simulink model "targetingLib"  (R2026b)
settings: Solver=VariableStepAuto
undefined symbols (not defined in the file or in its folder): maxval_sc, minval_sc, modval, samptime, Slope1, Slope2, threshold_add
libraries: hdlsllib x57, simulink x19, simulink_extras x11, dspsigops x2, sl_signal_attributes x2
(part 2 of 3)

== system targetingLib/Energy Detector/CalibrationPacketisation/Detect Overflow1 ==
  note: Throw away if not ready.
      | Assume will always be ready due to low rates.
  Ready : Inport
  Valid : Inport  Port=2
  EOB : Inport  Port=3
  AND1 : Logic  IconShape=distinctive  AllPortsSameDT=off  OutDataTypeStr=boolean
  AND2 : Logic  IconShape=distinctive  AllPortsSameDT=off  OutDataTypeStr=boolean
  Delay : Delay  DelayLength=1
  NOT : Logic  Operator=NOT  IconShape=distinctive  AllPortsSameDT=off  OutDataTypeStr=boolean
  Reset on next burst : simulink_extras/Flip Flops/S-R Flip-Flop  initial_condition=0
  Start of Burst : Subsystem
  Terminator : Terminator
  ValidOut : Outport
  OverflowOut : Outport  Port=2
  wires:
  AND1/1 -> ValidOut/1
  Ready/1 -> AND1/2, NOT/1
  Valid/1 -> AND2/2, Start of Burst/1(Valid), AND1/1  "Valid"
  NOT/1 -> AND2/1
  EOB/1 -> Start of Burst/2(EOB)  "EOB"
  Start of Burst/1(SOB) -> Reset on next burst/2
  AND2/1 -> Delay/1
  Reset on next burst/1 -> OverflowOut/1
  Reset on next burst/2 -> Terminator/1
  Delay/1 -> Reset on next burst/1

== system targetingLib/Energy Detector/Detect Overflow/Start of Burst ==
  Valid : Inport
  EOB : Inport  Port=2
  Detect Increase : simulink/Logic and Bit Operations/Detect Increase  vinit=0.0  OutDataTypeStr=boolean
  S-R Flip-Flop : simulink_extras/Flip Flops/S-R Flip-Flop  initial_condition=0
  Terminator : Terminator
  SOB : Outport
  wires:
  S-R Flip-Flop/1 -> Detect Increase/1
  EOB/1 -> S-R Flip-Flop/2
  S-R Flip-Flop/2 -> Terminator/1
  Detect Increase/1 -> SOB/1  "SOB"
  Valid/1 -> S-R Flip-Flop/1

== system targetingLib/Energy Detector/Energy Detector/Create Meta Data Stream ==
  note: 16 bits of pulse count
  note: Save pulse detection metadata as a uint32
  note: 16 bits of peak energy
  Energy : Inport
  Triggered_Data_Bus_Out : Inport  Port=2
  AND : Logic  IconShape=distinctive  AllPortsSameDT=off  OutDataTypeStr=boolean
  Bit Concat : hdlsllib/Logic and Bit Operations/Bit Concat  numInputs=2
  Bit Slice : hdlsllib/Logic and Bit Operations/Bit Slice  lidx=31  ridx=0
  Bit Slice1 : hdlsllib/Logic and Bit Operations/Bit Slice  lidx=63  ridx=32
  Bus Selector1 : BusSelector  OutputSignals=valid
  Bus Selector2 : BusSelector  OutputSignals=sampleTimestamp
  Bus Selector3 : BusSelector  OutputSignals=EndOfBurst
  Compare To Constant : simulink/Logic and Bit Operations/Compare To Constant  relop===  const=0  OutDataTypeStr=boolean
  Delay1 : Delay  DelayLength=1
  Delay2 : Delay  DelayLength=1
  Delay3 : Delay
  Delay4 : Delay  DelayLength=1
  Detect Increase : simulink/Logic and Bit Operations/Detect Increase  vinit=0.0  OutDataTypeStr=boolean
  Detected Pulse Length Counter : Subsystem
  Float Typecast1 : FloatTypecast
  Multiport Switch : MultiPortSwitch  DataPortOrder=Zero-based contiguous  zeroidx=on  SaturateOnIntegerOverflow=off  InputSameDT=off
  Multiport Controller : Subsystem
  Peak pulse energy : Subsystem
  Meta_Data_Data : Outport
  Meta_Data_Valid : Outport  Port=2
  wires:
  Triggered_Data_Bus_Out/1 -> Bus Selector3/1, Bus Selector1/1, Bus Selector2/1
  Energy/1 -> Peak pulse energy/1(energy)
  Float Typecast1/1 -> Bit Concat/1
  Bus Selector3/1 -> Detect Increase/1  "<EndOfBurst>"
  Detected Pulse Length Counter/1(count) -> Bit Concat/2
  Peak pulse energy/1(peak) -> Float Typecast1/1
  Detect Increase/1 -> Delay2/1
  Bus Selector1/1 -> Peak pulse energy/3(valid), Detected Pulse Length Counter/2(valid)  "<valid>"
  Bus Selector2/1 -> Bit Slice1/1, Bit Slice/1  "<sampleTimestamp>"
  Multiport Switch/1 -> Meta_Data_Data/1
  Bit Concat/1 -> Multiport Switch/2
  Bit Slice1/1 -> Delay1/1
  Bit Slice/1 -> Delay3/1
  Delay1/1 -> Multiport Switch/3
  Delay3/1 -> Multiport Switch/4
  Delay2/1 -> Multiport Controller/1(EoB_Asserted)
  Multiport Controller/2(count) -> Compare To Constant/1, Multiport Switch/1
  Multiport Controller/1(valid_out) -> AND/2, Meta_Data_Valid/1
  [PeakRst] -> Detected Pulse Length Counter/1(rst), Peak pulse energy/2(rst)
  Compare To Constant/1 -> AND/1
  AND/1 -> Delay4/1
  Delay4/1 -> [PeakRst]

== system targetingLib/Energy Detector/Energy Detector/Energy Detector ==
  DataBusIn : Inport
  WindowLength : Inport  Port=2
  AdaptiveThreshold : Inport  Port=3
  AdaptiveEndThreshold : Inport  Port=4
  AdaptiveThresholdScaler : Inport  Port=5
  FixedThreshold : Inport  Port=6
  Bus Selector : BusSelector  OutputSignals=EndOfBurst
  Delay : Delay  DelayLength=1
  Signal Detection : Subsystem
  Energy : Outport
  DataBusOut : Outport  Port=2
  Triggered : Outport  Port=3
  CalibrationOut : Outport  Port=4
  wires:
  WindowLength/1 -> Signal Detection/3(delay_len)  "WindowLength"
  FixedThreshold/1 -> Signal Detection/4(fix_threshold_in)  "FixedThreshold"
  DataBusIn/1 -> Signal Detection/2(data_bus_in)
  Signal Detection/3(Trigger_Out) -> Triggered/1
  Signal Detection/4(Energy_out) -> Energy/1
  Signal Detection/2(FT_Data_Out) -> CalibrationOut/1
  Delay/1 -> Signal Detection/1(rst)
  Signal Detection/1(Data_Bus_Out) -> Bus Selector/1, DataBusOut/1
  AdaptiveThreshold/1 -> Signal Detection/5(adp_threshold_in)  "AdaptiveThreshold"
  AdaptiveThresholdScaler/1 -> Signal Detection/7(adp_normalizer)  "AdaptiveThresholdScaler"
  AdaptiveEndThreshold/1 -> Signal Detection/6(adp_end_threshold_in)  "AdaptiveEndThreshold"
  Bus Selector/1 -> Delay/1  "<EndOfBurst>"

== system targetingLib/Energy Detector/Energy Detector/Triggered Burst Formatting ==
  note: Reset state when Burst from Radio ends (EOB from Radio)
  note: Handle trigger not in sync with Valid by holding EOB high
  note: When data is valid and trigger is true, out is valid
  note: Trigger is de-asserted, end the burst.
  Data_Bus_In : Inport
  Trigger : Inport  Port=2
  AND : Logic  IconShape=distinctive  AllPortsSameDT=off  OutDataTypeStr=boolean
  AND1 : Logic  IconShape=distinctive  AllPortsSameDT=off  OutDataTypeStr=boolean
  Bus Selector : BusSelector  OutputSignals=data,sampleTimestamp,valid,EndOfBurst
  Bus Selector1 : BusSelector  OutputSignals=data,sampleTimestamp
  Data Bus : BusCreator  Inputs=4
  Delay1 : Delay
  Delay2 : Delay
  Delay3 : Delay  DelayLength=1
  Delay4 : Delay  DelayLength=1
  Delay5 : Delay
  End of trigger : simulink/Logic and Bit Operations/Detect Decrease  vinit=0.0  OutDataTypeStr=boolean
  EndedByRadio : Logic  IconShape=distinctive  AllPortsSameDT=off  OutDataTypeStr=boolean
  OR : Logic  Operator=OR  IconShape=distinctive  AllPortsSameDT=off  OutDataTypeStr=boolean
  S-R Flip-Flop : simulink_extras/Flip Flops/S-R Flip-Flop  initial_condition=0
  Sideband Bus : BusCreator  Inputs=2
  Terminator : Terminator
  Data_Bus_Out : Outport
  Reset_Out : Outport  Port=2
  wires:
  Trigger/1 -> EndedByRadio/1, End of trigger/1, AND/1
  AND/1 -> Delay1/1
  End of trigger/1 -> OR/1
  Delay1/1 -> Data Bus/3, AND1/1  "valid"
  OR/1 -> Delay4/1
  S-R Flip-Flop/1 -> AND1/2, Data Bus/4  "EndOfBurst"
  AND1/1 -> Delay3/1
  S-R Flip-Flop/2 -> Terminator/1
  Delay3/1 -> S-R Flip-Flop/2
  Delay4/1 -> S-R Flip-Flop/1
  Delay5/1 -> Reset_Out/1
  Data_Bus_In/1 -> Bus Selector/1
  Bus Selector/3 -> AND/2  "<valid>"
  Bus Selector/4 -> Delay5/1, EndedByRadio/2  "<EndOfBurst>"
  Bus Selector/1 -> Sideband Bus/1  "<data>"
  Bus Selector/2 -> Sideband Bus/2  "<sampleTimestamp>"
  Sideband Bus/1 -> Delay2/1  "SidebandBus"
  Delay2/1 -> Bus Selector1/1
  Bus Selector1/1 -> Data Bus/1  "<data>"
  Bus Selector1/2 -> Data Bus/2  "<sampleTimestamp>"
  Data Bus/1 -> Data_Bus_Out/1
  EndedByRadio/1 -> OR/2

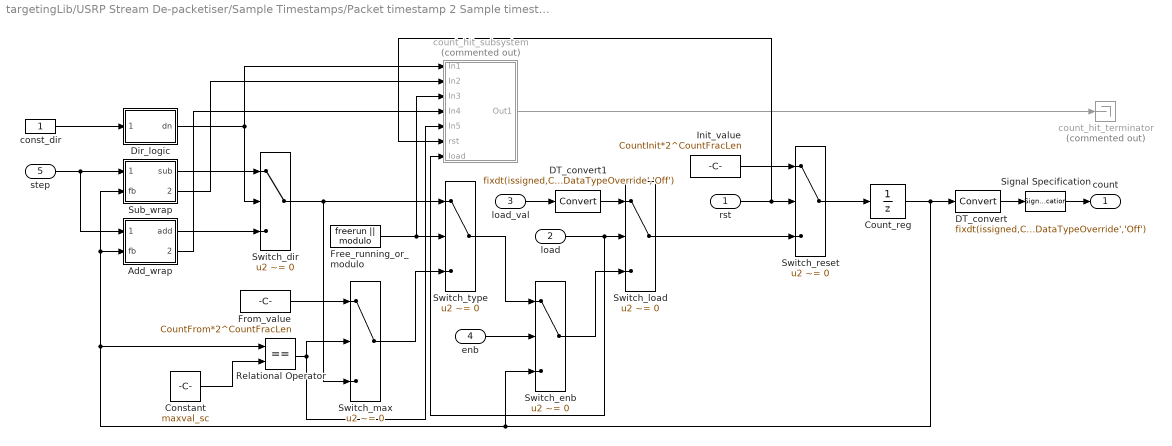
== system targetingLib/USRP Stream De-packetiser/Sample Timestamps/Packet timestamp 2 Sample timestamp ==
  rst : Inport  OutDataTypeStr=boolean  PortDimensions=1
  load : Inport  Port=2  OutDataTypeStr=boolean  PortDimensions=1
  load_val : Inport  Port=3  OutDataTypeStr=fixdt(issigned,CountWordLen,CountFracLen,'DataTypeOverride','Off')  PortDimensions=1
  enb : Inport  Port=4  OutDataTypeStr=boolean  PortDimensions=1
  step : Inport  Port=5  OutDataTypeStr=uint64  PortDimensions=1
  Add_wrap : Subsystem
  Constant : Constant  Value=maxval_sc  OutDataTypeStr=fixdt(issigned,CountWordLen,0,'DataTypeOverride','Off')  SampleTime=-1
  Count_reg : UnitDelay  InitialCondition=CountInit*2^CountFracLen  SampleTime=samptime
  DT_convert : DataTypeConversion  OutDataTypeStr=fixdt(issigned,CountWordLen,CountFracLen,'DataTypeOverride','Off')  ConvertRealWorld=Stored Integer (SI)  SaturateOnIntegerOverflow=off  RndMeth=Floor
  DT_convert1 : DataTypeConversion  OutDataTypeStr=fixdt(issigned,CountWordLen,0,'DataTypeOverride','Off')  ConvertRealWorld=Stored Integer (SI)  SaturateOnIntegerOverflow=off  RndMeth=Floor
  Dir_logic : Subsystem
  Free_running_or_modulo : Constant  Value=freerun || modulo  OutDataTypeStr=boolean  SampleTime=-1
  From_value : Constant  Value=CountFrom*2^CountFracLen  OutDataTypeStr=fixdt(issigned,CountWordLen, 0,'DataTypeOverride','Off')  SampleTime=-1
  Init_value : Constant  Value=CountInit*2^CountFracLen  OutDataTypeStr=fixdt(issigned,CountWordLen, 0,'DataTypeOverride','Off')  SampleTime=-1
  Relational Operator : RelationalOperator  Operator===  OutDataTypeStr=boolean  RndMeth=Simplest  InputSameDT=off
  Signal Specification : SignalSpecification  Dimensions=1
  Sub_wrap : Subsystem
  Switch_dir : Switch  Criteria=u2 ~= 0  SaturateOnIntegerOverflow=off  InputSameDT=off
  Switch_enb : Switch  Criteria=u2 ~= 0  SaturateOnIntegerOverflow=off  InputSameDT=off
  Switch_load : Switch  Criteria=u2 ~= 0  SaturateOnIntegerOverflow=off  InputSameDT=off
  Switch_max : Switch  Criteria=u2 ~= 0  SaturateOnIntegerOverflow=off  InputSameDT=off
  Switch_reset : Switch  Criteria=u2 ~= 0  OutDataTypeStr=fixdt(issigned,CountWordLen, 0,'DataTypeOverride','Off')  SaturateOnIntegerOverflow=off  InputSameDT=off
  Switch_type : Switch  Criteria=u2 ~= 0  SaturateOnIntegerOverflow=off  InputSameDT=off
  const_dir : Constant  OutDataTypeStr=boolean  SampleTime=-1
  count_hit_subsystem : Subsystem  Commented=on
  count_hit_terminator : Terminator  Commented=on
  count : Outport  OutDataTypeStr=uint64  VectorParamsAs1DForOutWhenUnconnected=off
  wires:
  count_hit_subsystem/1(Out1) -> count_hit_terminator/1
  Add_wrap/2(count_hit) -> count_hit_subsystem/4(In4)
  Sub_wrap/2(count_hit) -> count_hit_subsystem/2(In2)
  Relational Operator/1 -> count_hit_subsystem/5(In5), Switch_max/2
  Constant/1 -> Relational Operator/2
  Switch_dir/1 -> Switch_type/1, Switch_max/3
  Init_value/1 -> Switch_reset/1
  rst/1 -> Switch_reset/2, count_hit_subsystem/6(rst)
  Switch_reset/1 -> Count_reg/1
  Count_reg/1 -> Switch_enb/3, Sub_wrap/2(fb), Add_wrap/2(fb), Relational Operator/1, DT_convert/1
  Switch_load/1 -> Switch_reset/3
  load/1 -> Switch_load/2, count_hit_subsystem/7(load)
  load_val/1 -> DT_convert1/1
  Switch_enb/1 -> Switch_load/3
  enb/1 -> Switch_enb/2
  const_dir/1 -> Dir_logic/1(dir_port)
  step/1 -> Add_wrap/1(step), Sub_wrap/1(step)
  Switch_type/1 -> Switch_enb/1
  From_value/1 -> Switch_max/1
  Switch_max/1 -> Switch_type/3
  Free_running_or_modulo/1 -> Switch_type/2, count_hit_subsystem/3(In3)
  DT_convert/1 -> Signal Specification/1
  Add_wrap/1(add) -> Switch_dir/3
  Sub_wrap/1(sub) -> Switch_dir/1
  Dir_logic/1(dn) -> Switch_dir/2, count_hit_subsystem/1(In1)
  DT_convert1/1 -> Switch_load/1
  Signal Specification/1 -> count/1

== system targetingLib/Energy Detector/CalibrationPacketisation/Detect Overflow/Start of Burst ==
  Valid : Inport
  EOB : Inport  Port=2
  Detect Increase : simulink/Logic and Bit Operations/Detect Increase  vinit=0.0  OutDataTypeStr=boolean
  S-R Flip-Flop : simulink_extras/Flip Flops/S-R Flip-Flop  initial_condition=0
  Terminator : Terminator
  SOB : Outport
  wires:
  S-R Flip-Flop/1 -> Detect Increase/1
  EOB/1 -> S-R Flip-Flop/2
  S-R Flip-Flop/2 -> Terminator/1
  Detect Increase/1 -> SOB/1  "SOB"
  Valid/1 -> S-R Flip-Flop/1

== system targetingLib/Energy Detector/CalibrationPacketisation/Detect Overflow1/Start of Burst ==
  Valid : Inport
  EOB : Inport  Port=2
  Detect Increase : simulink/Logic and Bit Operations/Detect Increase  vinit=0.0  OutDataTypeStr=boolean
  S-R Flip-Flop : simulink_extras/Flip Flops/S-R Flip-Flop  initial_condition=0
  Terminator : Terminator
  SOB : Outport
  wires:
  S-R Flip-Flop/1 -> Detect Increase/1
  EOB/1 -> S-R Flip-Flop/2
  S-R Flip-Flop/2 -> Terminator/1
  Detect Increase/1 -> SOB/1  "SOB"
  Valid/1 -> S-R Flip-Flop/1

== system targetingLib/Energy Detector/Energy Detector/Create Meta Data Stream/Detected Pulse Length Counter ==
  note: when overflow, set count to zero
  rst : Inport
  valid : Inport  Port=2
  Constant : Constant  Value=0  OutDataTypeStr=Inherit: Inherit via back propagation
  HDL Counter : hdlsllib/Sources/HDL Counter  CountType=Free running  CountInit=0  CountStep=1  CountMax=25  CountFromType=Initial value  CountFrom=0  CountResetPort=on  CountLoadPort=off  CountEnbPort=on  CountDirPort=off  CountHitOutputPort=on  CountDataType=Unsigned  CountWordLen=16  CountFracLen=0  CountSampTime=1
  Multiport Switch : MultiPortSwitch  DataPortOrder=Zero-based contiguous  Inputs=2  zeroidx=on  SaturateOnIntegerOverflow=off  InputSameDT=off
  S-R Flip-Flop : simulink_extras/Flip Flops/S-R Flip-Flop  initial_condition=0
  Terminator : Terminator
  count : Outport
  wires:
  valid/1 -> HDL Counter/2
  HDL Counter/2 -> S-R Flip-Flop/1
  rst/1 -> S-R Flip-Flop/2, HDL Counter/1
  S-R Flip-Flop/2 -> Terminator/1
  S-R Flip-Flop/1 -> Multiport Switch/1
  HDL Counter/1 -> Multiport Switch/2
  Constant/1 -> Multiport Switch/3
  Multiport Switch/1 -> count/1

== system targetingLib/Energy Detector/Energy Detector/Create Meta Data Stream/Multiport Controller ==
  note: On EoB (end of detected pulse), hold metadata valid high for three cycles and iterate the multiport switch index
  EoB_Asserted : Inport
  Delay : Delay  DelayLength=1  InputProcessing=Columns as channels (frame based)
  HDL Counter : hdlsllib/Sources/HDL Counter  CountType=Count limited  CountInit=0  CountStep=1  CountMax=2  CountFromType=Initial value  CountFrom=0  CountResetPort=off  CountLoadPort=off  CountEnbPort=on  CountDirPort=off  CountHitOutputPort=on  CountDataType=Unsigned  CountWordLen=2  CountFracLen=0  CountSampTime=1
  S-R Flip-Flop : simulink_extras/Flip Flops/S-R Flip-Flop  initial_condition=0
  Terminator : Terminator
  valid_out : Outport
  count : Outport  Port=2
  wires:
  HDL Counter/2 -> Delay/1
  S-R Flip-Flop/1 -> valid_out/1, HDL Counter/1
  S-R Flip-Flop/2 -> Terminator/1
  EoB_Asserted/1 -> S-R Flip-Flop/1
  HDL Counter/1 -> count/1
  Delay/1 -> S-R Flip-Flop/2

== system targetingLib/Energy Detector/Energy Detector/Create Meta Data Stream/Peak pulse energy ==
  energy : Inport
  rst : Inport  Port=2
  valid : Inport  Port=3
  AND : Logic  Inputs=3  IconShape=distinctive  AllPortsSameDT=off  OutDataTypeStr=boolean
  AND1 : Logic  IconShape=distinctive  AllPortsSameDT=off  OutDataTypeStr=boolean
  Constant : Constant  Value=0  OutDataTypeStr=Inherit: Inherit via back propagation
  Delay{1..3,5} (4 alike) : Delay  DelayLength=1
  GreaterThan : RelationalOperator  Operator=>  OutDataTypeStr=boolean  RndMeth=Simplest  InputSameDT=off
  GreaterThan1 : RelationalOperator  Operator=>  OutDataTypeStr=boolean  RndMeth=Simplest  InputSameDT=off
  Multiport Switch : MultiPortSwitch  DataPortOrder=Zero-based contiguous  Inputs=2  zeroidx=on  SaturateOnIntegerOverflow=off  InputSameDT=off
  NOT : Logic  Operator=NOT  IconShape=distinctive  AllPortsSameDT=off  OutDataTypeStr=boolean
  NOT1 : Logic  Operator=NOT  IconShape=distinctive  AllPortsSameDT=off  OutDataTypeStr=boolean
  OR : Logic  Operator=OR  IconShape=distinctive  AllPortsSameDT=off  OutDataTypeStr=boolean
  Sample and Hold : dspsigops/Sample and Hold  trig=Falling edge  initCond=0  latchinput=off
  peak : Outport
  wires:
  Sample and Hold/1 -> Delay1/1, peak/1  "Held_Peak_Energy"
  rst/1 -> NOT/1, Delay2/1
  energy/1 -> Multiport Switch/3
  Constant/1 -> Multiport Switch/2
  OR/1 -> Delay5/1
  Delay1/1 -> GreaterThan/2
  valid/1 -> AND/3
  AND/1 -> Multiport Switch/1
  NOT/1 -> AND/2
  NOT1/1 -> AND/1
  Multiport Switch/1 -> Delay3/1, GreaterThan/1, GreaterThan1/1  "S&H_In_z-1"
  Delay2/1 -> OR/1, NOT1/1
  Delay5/1 -> Sample and Hold/Trigger  "S&H_Trigger"
  Delay3/1 -> GreaterThan1/2, Sample and Hold/1  "S&H_In"
  GreaterThan/1 -> AND1/1
  AND1/1 -> OR/2
  GreaterThan1/1 -> AND1/2

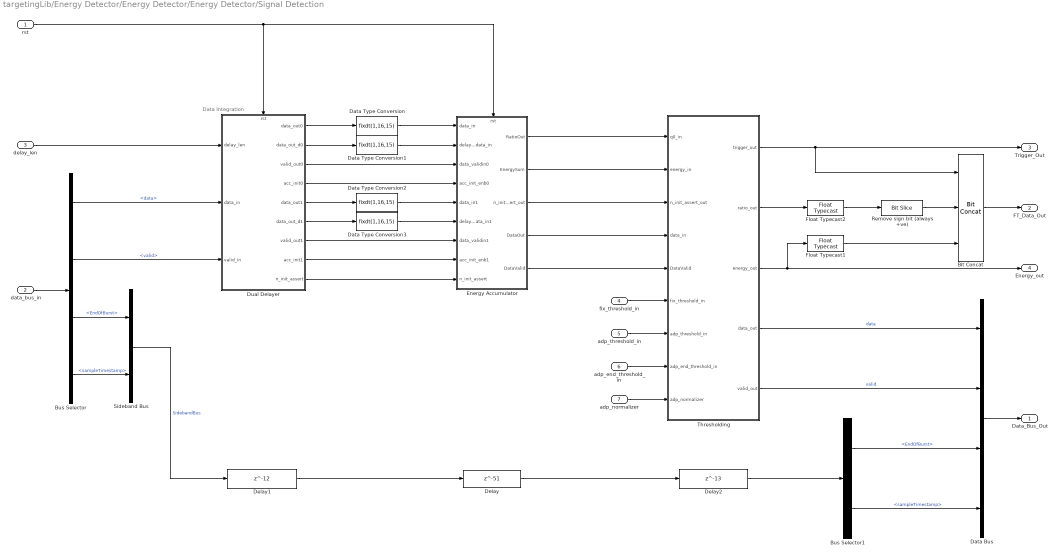
== system targetingLib/Energy Detector/Energy Detector/Energy Detector/Signal Detection ==
  note: Data Integration
  rst : Inport
  data_bus_in : Inport  Port=2
  delay_len : Inport  Port=3
  fix_threshold_in : Inport  Port=4
  adp_threshold_in : Inport  Port=5
  adp_end_threshold_in : Inport  Port=6
  adp_normalizer : Inport  Port=7
  Bit Concat : hdlsllib/Logic and Bit Operations/Bit Concat  numInputs=3
  Bus Selector : BusSelector  OutputSignals=data,valid,EndOfBurst,sampleTimestamp
  Bus Selector1 : BusSelector  OutputSignals=EndOfBurst,sampleTimestamp
  Data Bus : BusCreator  Inputs=4
  Data Type Conversion{,1..3} (4 alike) : DataTypeConversion  OutDataTypeStr=fixdt(1,16,15)  ConvertRealWorld=Stored Integer (SI)  SaturateOnIntegerOverflow=off  RndMeth=Floor
  Delay : Delay  DelayLength=51
  Delay1 : Delay  DelayLength=12
  Delay2 : Delay  DelayLength=13
  Dual Delayer : Subsystem
      settings: PortSchema="{\"entries\":[{\"content\":{\"sides\":[{\"content\":{\"connectorIds\":[\"In1\",\"In2\",\"In3\"]},\"type\":\"ConnectorPlacement.EquallySpacedRectSide\",\"uuid\":\"1990f724-ce81-4930-8303-ca4574d8597a\"},{\"content\":{\"connectorIds\":[\"Out1\",\"Out2\",\"Out3\",\"Out4\",\"Out5\",\"Out6\",\"Out7\",\"Out8\",\"Out9\"],\"side\":\"RIGHT\"},\"type\":\"ConnectorPlacement.EquallySpacedRectSide\",\"uuid\":\"07aa7081-9df9-4b7b-99cf-18a69e24a9dd\"},{\"content\":{\"connectorIds\":[\"In4\"],\"side\":\"TOP\"},\"type\":\"ConnectorPlacement.EquallySpacedRectSide\",\"uuid\":\"c539866f-8e74-4e5e-8c91-443fc7644965\"}]},\"type\":\"ConnectorPlacement.EquallySpacedConnector\",\"uuid\":\"51e43d27-2fb9-458c-abe5-78da9f37cda7\"}],\"packageUris\":[\"http://schema.mathworks.com/mf0/Connector/R2020b\"],\"version\":\"1.0\"}"
  Energy Accumulator : Subsystem
      settings: PortSchema="{\"entries\":[{\"content\":{\"sides\":[{\"content\":{\"connectorIds\":[\"In1\",\"In2\",\"In3\",\"In4\",\"In5\",\"In6\",\"In7\",\"In8\",\"In9\"]},\"type\":\"ConnectorPlacement.EquallySpacedRectSide\",\"uuid\":\"77e2cb86-5f48-4a80-b1b2-d7609ed2078a\"},{\"content\":{\"connectorIds\":[\"Out1\",\"Out2\",\"Out3\",\"Out4\",\"Out5\"],\"side\":\"RIGHT\"},\"type\":\"ConnectorPlacement.EquallySpacedRectSide\",\"uuid\":\"c00c0dae-d92b-414e-ab86-0e0e4d62d9d4\"},{\"content\":{\"connectorIds\":[\"In10\"],\"side\":\"TOP\"},\"type\":\"ConnectorPlacement.EquallySpacedRectSide\",\"uuid\":\"ff834e34-3849-439a-94b9-46a3f8fae257\"},{\"content\":{\"side\":\"BOTTOM\"},\"type\":\"ConnectorPlacement.EquallySpacedRectSide\",\"uuid\":\"b228cde8-67b0-4813-8a7b-4abc66a019f0\"}]},\"type\":\"ConnectorPlacement.EquallySpacedConnector\",\"uuid\":\"f3253208-8d8b-42fb-83fa-c8e1dc6b6bcd\"}],\"packageUris\":[\"http://schema.mathworks.com/mf0/Connector/R2020b\"],\"version\":\"1.0\"}"
  Float Typecast1 : FloatTypecast
  Float Typecast2 : FloatTypecast
  Remove sign bit (always +ve) : hdlsllib/Logic and Bit Operations/Bit Slice  lidx=14  ridx=0
  Sideband Bus : BusCreator  Inputs=2
  Thresholding : Subsystem
  Data_Bus_Out : Outport
  FT_Data_Out : Outport  Port=2
  Trigger_Out : Outport  Port=3
  Energy_out : Outport  Port=4
  wires:
  Dual Delayer/8(acc_init1) -> Energy Accumulator/8(acc_init_enb1)
  Data Type Conversion/1 -> Energy Accumulator/1(data_in)
  Dual Delayer/6(data_out_d1) -> Data Type Conversion3/1
  Dual Delayer/4(acc_init0) -> Energy Accumulator/4(acc_init_enb0)
  Energy Accumulator/3(n_init_assert_out) -> Thresholding/3(n_init_assert_out)
  Dual Delayer/5(data_out1) -> Data Type Conversion2/1
  fix_threshold_in/1 -> Thresholding/6(fix_threshold_in)
  Thresholding/4(data_out) -> Data Bus/1  "data"
  adp_threshold_in/1 -> Thresholding/7(adp_threshold_in)
  Data Type Conversion3/1 -> Energy Accumulator/6(delay_data_in1)
  delay_len/1 -> Dual Delayer/1(delay_len)
  Dual Delayer/1(data_out0) -> Data Type Conversion/1
  Energy Accumulator/2(EnergySum) -> Thresholding/2(energy_in)
  rst/1 -> Energy Accumulator/10(rst), Dual Delayer/4(rst)
  Data Type Conversion2/1 -> Energy Accumulator/5(data_in1)
  Thresholding/5(valid_out) -> Data Bus/2  "valid"
  Energy Accumulator/1(RatioOut) -> Thresholding/1(q0_in)
  Data Type Conversion1/1 -> Energy Accumulator/2(delay_data_in)
  Dual Delayer/9(n_init_assert) -> Energy Accumulator/9(n_init_assert)
  Energy Accumulator/5(DataValid) -> Thresholding/5(DataValid)
  adp_normalizer/1 -> Thresholding/9(adp_normalizer)
  Thresholding/1(trigger_out) -> Trigger_Out/1, Bit Concat/1
  Dual Delayer/7(valid_out1) -> Energy Accumulator/7(data_validin1)
  Dual Delayer/2(data_out_d0) -> Data Type Conversion1/1
  Dual Delayer/3(valid_out0) -> Energy Accumulator/3(data_validin0)
  Thresholding/3(energy_out) -> Energy_out/1, Float Typecast1/1
  Energy Accumulator/4(DataOut) -> Thresholding/4(data_in)
  Bit Concat/1 -> FT_Data_Out/1
  Delay1/1 -> Delay/1
  Delay/1 -> Delay2/1
  adp_end_threshold_in/1 -> Thresholding/8(adp_end_threshold_in)
  Float Typecast2/1 -> Remove sign bit (always +ve)/1
  Remove sign bit (always +ve)/1 -> Bit Concat/2
  Thresholding/2(ratio_out) -> Float Typecast2/1
  Float Typecast1/1 -> Bit Concat/3
  data_bus_in/1 -> Bus Selector/1
  Bus Selector/1 -> Dual Delayer/2(data_in)  "<data>"
  Bus Selector/2 -> Dual Delayer/3(valid_in)  "<valid>"
  Bus Selector/3 -> Sideband Bus/1  "<EndOfBurst>"
  Bus Selector/4 -> Sideband Bus/2  "<sampleTimestamp>"
  Sideband Bus/1 -> Delay1/1  "SidebandBus"
  Delay2/1 -> Bus Selector1/1
  Bus Selector1/1 -> Data Bus/3  "<EndOfBurst>"
  Bus Selector1/2 -> Data Bus/4  "<sampleTimestamp>"
  Data Bus/1 -> Data_Bus_Out/1

== system targetingLib/USRP Stream De-packetiser/Sample Timestamps/Packet timestamp 2 Sample timestamp/Add_wrap ==
  step : Inport
  fb : Inport  Port=2
  Add : Sum  OutDataTypeStr=Inherit: Same as accumulator  AccumDataTypeStr=fixdt(issigned,CountWordLen+1,0)
  Compare To Constant : hdlsllib/Logic and Bit Operations/Compare To Constant  relop=>  const=threshold_add  OutDataTypeStr=boolean
  Mod_value : Constant  Value=modval  OutDataTypeStr=fixdt(0,CountWordLen+1,0,'DataTypeOverride','Off')  SampleTime=-1
  Switch_wrap : Switch  Criteria=u2 > Threshold  Threshold=threshold_add  OutDataTypeStr=fixdt(issigned,CountWordLen,0,'DataTypeOverride','Off')  SaturateOnIntegerOverflow=off  InputSameDT=off
  Wrap : Sum  Inputs=-+  OutDataTypeStr=Inherit: Same as accumulator  AccumDataTypeStr=fixdt(1,CountWordLen+3,0)
  add : Outport  VectorParamsAs1DForOutWhenUnconnected=off
  count_hit : Outport  Port=2  VectorParamsAs1DForOutWhenUnconnected=off
  wires:
  Compare To Constant/1 -> count_hit/1
  step/1 -> Add/1
  Switch_wrap/1 -> add/1
  fb/1 -> Add/2
  Wrap/1 -> Switch_wrap/1
  Add/1 -> Wrap/2, Switch_wrap/2, Switch_wrap/3, Compare To Constant/1
  Mod_value/1 -> Wrap/1

== system targetingLib/USRP Stream De-packetiser/Sample Timestamps/Packet timestamp 2 Sample timestamp/Dir_logic ==
  dir_port : Inport  OutDataTypeStr=boolean
  Logical Operator : Logic  Operator=XOR  AllPortsSameDT=off  OutDataTypeStr=boolean
  Pos_step : Constant  Value=(sign(CountStep) == 1)  OutDataTypeStr=boolean  SampleTime=-1
  dn : Outport  VectorParamsAs1DForOutWhenUnconnected=off
  wires:
  Logical Operator/1 -> dn/1
  Pos_step/1 -> Logical Operator/2
  dir_port/1 -> Logical Operator/1

== system targetingLib/USRP Stream De-packetiser/Sample Timestamps/Packet timestamp 2 Sample timestamp/Sub_wrap ==
  step : Inport
  fb : Inport  Port=2
  Add : Sum  Inputs=-+  OutDataTypeStr=Inherit: Same as accumulator  AccumDataTypeStr=fixdt(1,CountWordLen+1,0)
  Compare To Constant : hdlsllib/Logic and Bit Operations/Compare To Constant  relop=<  const=minval_sc  OutDataTypeStr=boolean
  Mod_value : Constant  Value=modval  OutDataTypeStr=fixdt(0,CountWordLen+1,0,'DataTypeOverride','Off')  SampleTime=-1
  Switch_wrap : Switch  Threshold=minval_sc  OutDataTypeStr=fixdt(issigned,CountWordLen,0,'DataTypeOverride','Off')  SaturateOnIntegerOverflow=off  InputSameDT=off
  Wrap : Sum  OutDataTypeStr=Inherit: Same as accumulator  AccumDataTypeStr=fixdt(1,CountWordLen+3,0)
  sub : Outport  VectorParamsAs1DForOutWhenUnconnected=off
  count_hit : Outport  Port=2  VectorParamsAs1DForOutWhenUnconnected=off
  wires:
  Compare To Constant/1 -> count_hit/1
  fb/1 -> Add/2
  Switch_wrap/1 -> sub/1
  step/1 -> Add/1
  Add/1 -> Wrap/1, Switch_wrap/1, Switch_wrap/2, Compare To Constant/1
  Mod_value/1 -> Wrap/2
  Wrap/1 -> Switch_wrap/3

== system targetingLib/USRP Stream De-packetiser/Sample Timestamps/Packet timestamp 2 Sample timestamp/count_hit_subsystem ==
  In1 : Inport
  In2 : Inport  Port=2
  In3 : Inport  Port=3
  In4 : Inport  Port=4
  In5 : Inport  Port=5
  rst : Inport  Port=6
  load : Inport  Port=7
  Constant : Constant  Value=0  OutDataTypeStr=boolean  SampleTime=-1
  Logical Operator : Logic  Operator=OR  AllPortsSameDT=off  OutDataTypeStr=boolean
  Logical Operator1 : Logic  Operator=OR  AllPortsSameDT=off  OutDataTypeStr=boolean
  Switch : Switch  Criteria=u2 ~= 0  SaturateOnIntegerOverflow=off  InputSameDT=off
  Switch1 : Switch  Criteria=u2 ~= 0  SaturateOnIntegerOverflow=off  InputSameDT=off
  Switch2 : Switch  Criteria=u2 ~= 0  SaturateOnIntegerOverflow=off  InputSameDT=off
  Out1 : Outport
  wires:
  In4/1 -> Switch/3
  Switch/1 -> Logical Operator/1, Switch1/1
  rst/1 -> Logical Operator1/1
  load/1 -> Logical Operator1/2
  Constant/1 -> Switch2/1
  Logical Operator1/1 -> Switch2/2
  Switch2/1 -> Out1/1
  In1/1 -> Switch/2
  In5/1 -> Logical Operator/2
  In3/1 -> Switch1/2
  Switch1/1 -> Switch2/3
  In2/1 -> Switch/1
  Logical Operator/1 -> Switch1/3

== system targetingLib/Energy Detector/Energy Detector/Energy Detector/Signal Detection/Dual Delayer ==
  delay_len : Inport
  data_in : Inport  Port=2
  valid_in : Inport  Port=3
  rst : Inport  Port=4
  Delay{,1..3} (4 alike) : Delay  DelayLength=6
  Logical Operator : Logic  AllPortsSameDT=off  OutDataTypeStr=boolean
  Variable Delayer0 : Subsystem  mask{depth=6}
  Variable Delayer1 : Subsystem  mask{depth=6}
  data_out0 : Outport
  data_out_d0 : Outport  Port=2
  valid_out0 : Outport  Port=3
  acc_init0 : Outport  Port=4
  data_out1 : Outport  Port=5
  data_out_d1 : Outport  Port=6
  valid_out1 : Outport  Port=7
  acc_init1 : Outport  Port=8
  n_init_assert : Outport  Port=9
  wires:
  Delay3/1 -> data_out0/1
  Delay2/1 -> data_out_d0/1
  Delay1/1 -> valid_out0/1
  Delay/1 -> acc_init0/1
  Variable Delayer0/5(acc_init) -> Delay/1
  Variable Delayer0/3(valid_out) -> Delay1/1, Logical Operator/1
  Variable Delayer0/2(data_out_d) -> Delay2/1, Variable Delayer1/1(data_in)
  Variable Delayer0/1(data_out) -> Delay3/1
  Variable Delayer0/4(n_init_assert) -> Logical Operator/2
  delay_len/1 -> Variable Delayer1/3(delay_len), Variable Delayer0/3(delay_len)
  rst/1 -> Variable Delayer1/4(rst), Variable Delayer0/4(rst)
  Logical Operator/1 -> Variable Delayer1/2(valid_in)
  Variable Delayer1/2(data_out_d) -> data_out_d1/1
  Variable Delayer1/1(data_out) -> data_out1/1
  valid_in/1 -> Variable Delayer0/2(valid_in)
  Variable Delayer1/5(acc_init) -> acc_init1/1
  data_in/1 -> Variable Delayer0/1(data_in)
  Variable Delayer1/4(n_init_assert) -> n_init_assert/1
  Variable Delayer1/3(valid_out) -> valid_out1/1

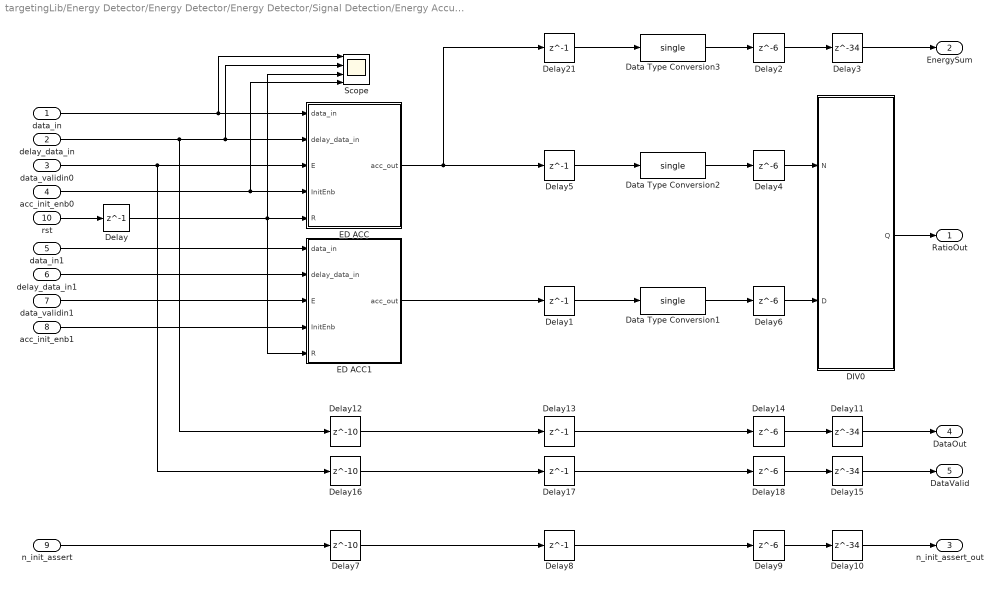
== system targetingLib/Energy Detector/Energy Detector/Energy Detector/Signal Detection/Energy Accumulator ==
  data_in : Inport
  delay_data_in : Inport  Port=2
  data_validin0 : Inport  Port=3
  acc_init_enb0 : Inport  Port=4
  data_in1 : Inport  Port=5
  delay_data_in1 : Inport  Port=6
  data_validin1 : Inport  Port=7
  acc_init_enb1 : Inport  Port=8
  n_init_assert : Inport  Port=9
  rst : Inport  Port=10
  DIV0 : Subsystem
  Data Type Conversion1 : DataTypeConversion  OutDataTypeStr=single  SaturateOnIntegerOverflow=off  RndMeth=Floor
  Data Type Conversion2 : DataTypeConversion  OutDataTypeStr=single  SaturateOnIntegerOverflow=off  RndMeth=Floor
  Data Type Conversion3 : DataTypeConversion  OutDataTypeStr=single  SaturateOnIntegerOverflow=off  RndMeth=Floor
  Delay{,1,5,8,13,17,21} (7 alike) : Delay  DelayLength=1
  Delay{3,10..11,15} (4 alike) : Delay  DelayLength=34
  Delay12 : Delay  DelayLength=10
  Delay{2,4,6,9,14,18} (6 alike) : Delay  DelayLength=6
  Delay16 : Delay  DelayLength=10
  Delay7 : Delay  DelayLength=10
  ED ACC : Subsystem  mask{bitwidth=45, bitwdith_low=22}
      mask prompts: bitwidth "Accumulator Bitwidth"; bitwdith_low "Lower Bitwdith"
  ED ACC1 : Subsystem  mask{bitwidth=45, bitwdith_low=22}
      mask prompts: bitwidth "Accumulator Bitwidth"; bitwdith_low "Lower Bitwdith"
  Scope : Scope  NumInputPorts=4
      settings: ActiveDisplayYMinimum=-0.62324905395507812  ActiveDisplayYMaximum=0.62480545043945312
  RatioOut : Outport
  EnergySum : Outport  Port=2
  n_init_assert_out : Outport  Port=3
  DataOut : Outport  Port=4
  DataValid : Outport  Port=5
  wires:
  Delay15/1 -> DataValid/1
  Delay11/1 -> DataOut/1
  Delay17/1 -> Delay18/1
  Delay16/1 -> Delay17/1
  Delay18/1 -> Delay15/1
  data_validin0/1 -> Delay16/1, ED ACC/3(E)
  delay_data_in/1 -> Delay12/1, ED ACC/2(delay_data_in), Scope/2
  Delay13/1 -> Delay14/1
  Delay12/1 -> Delay13/1
  Delay14/1 -> Delay11/1
  Delay10/1 -> n_init_assert_out/1
  Delay9/1 -> Delay10/1
  Delay8/1 -> Delay9/1
  Delay7/1 -> Delay8/1
  n_init_assert/1 -> Delay7/1
  Delay6/1 -> DIV0/2(D)
  Data Type Conversion1/1 -> Delay6/1
  Delay5/1 -> Data Type Conversion2/1
  Delay1/1 -> Data Type Conversion1/1
  Delay3/1 -> EnergySum/1
  Delay2/1 -> Delay3/1
  Data Type Conversion3/1 -> Delay2/1
  Delay4/1 -> DIV0/1(N)
  Data Type Conversion2/1 -> Delay4/1
  data_validin1/1 -> ED ACC1/3(E)
  rst/1 -> Delay/1
  data_in/1 -> ED ACC/1(data_in), Scope/1
  DIV0/1(Q) -> RatioOut/1
  acc_init_enb1/1 -> ED ACC1/4(InitEnb)
  delay_data_in1/1 -> ED ACC1/2(delay_data_in)
  acc_init_enb0/1 -> ED ACC/4(InitEnb), Scope/4
  data_in1/1 -> ED ACC1/1(data_in)
  ED ACC1/1(acc_out) -> Delay1/1
  ED ACC/1(acc_out) -> Delay21/1, Delay5/1
  Delay/1 -> ED ACC1/5(R), ED ACC/5(R), Scope/3
  Delay21/1 -> Data Type Conversion3/1

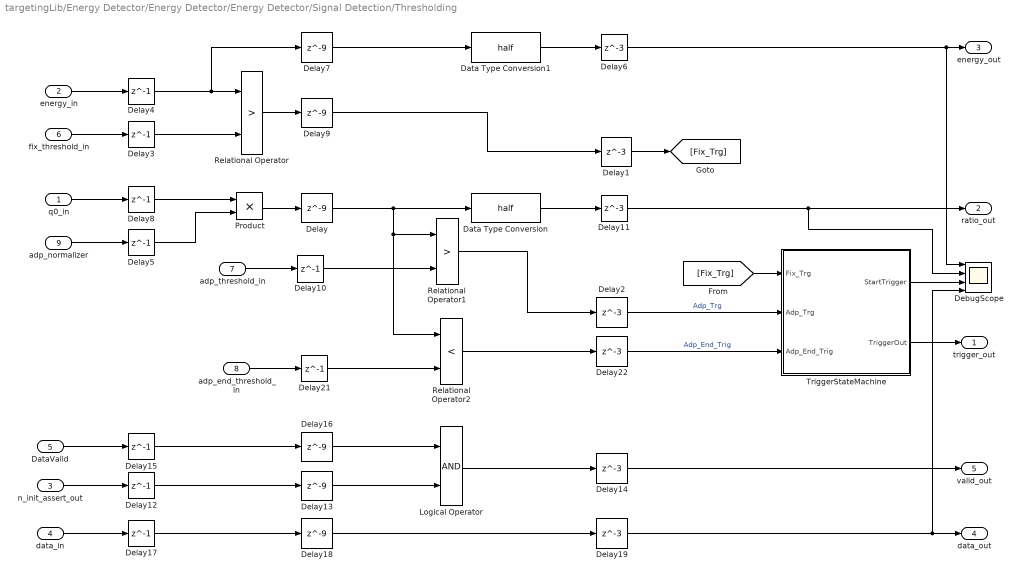
== system targetingLib/Energy Detector/Energy Detector/Energy Detector/Signal Detection/Thresholding ==
  q0_in : Inport
  energy_in : Inport  Port=2
  n_init_assert_out : Inport  Port=3
  data_in : Inport  Port=4
  DataValid : Inport  Port=5
  fix_threshold_in : Inport  Port=6
  adp_threshold_in : Inport  Port=7
  adp_end_threshold_in : Inport  Port=8
  adp_normalizer : Inport  Port=9
  Data Type Conversion : DataTypeConversion  OutDataTypeStr=half  SaturateOnIntegerOverflow=off  RndMeth=Floor
  Data Type Conversion1 : DataTypeConversion  OutDataTypeStr=half  SaturateOnIntegerOverflow=off  RndMeth=Floor
  DebugScope : Scope  NumInputPorts=4
      settings: ActiveDisplayString=3  ActiveDisplayYMinimum=-0.68578338623046875  ActiveDisplayYMaximum=1.1873092651367188
  Delay{,7,9,13,16,18} (6 alike) : Delay  DelayLength=9
  Delay{1..2,6,11,14,19,22} (7 alike) : Delay  DelayLength=3
  Delay{3..5,8,10,12,15,17,21} (9 alike) : Delay  DelayLength=1
  Logical Operator : Logic  AllPortsSameDT=off  OutDataTypeStr=boolean
  Product : Product
  Relational Operator : RelationalOperator  Operator=>  OutDataTypeStr=boolean  RndMeth=Simplest  InputSameDT=off
  Relational Operator1 : RelationalOperator  Operator=>  OutDataTypeStr=boolean  RndMeth=Simplest  InputSameDT=off
  Relational Operator2 : RelationalOperator  Operator=<  OutDataTypeStr=boolean  RndMeth=Simplest  InputSameDT=off
  TriggerStateMachine : Subsystem
  trigger_out : Outport
  ratio_out : Outport  Port=2
  energy_out : Outport  Port=3
  data_out : Outport  Port=4
  valid_out : Outport  Port=5
  wires:
  energy_in/1 -> Delay4/1
  Delay1/1 -> [Fix_Trg]
  Delay3/1 -> Relational Operator/2
  q0_in/1 -> Delay8/1
  Delay4/1 -> Relational Operator/1, Delay7/1
  fix_threshold_in/1 -> Delay3/1
  Data Type Conversion/1 -> Delay11/1
  Relational Operator/1 -> Delay9/1
  Relational Operator1/1 -> Delay2/1
  adp_threshold_in/1 -> Delay10/1
  Delay10/1 -> Relational Operator1/2
  adp_normalizer/1 -> Delay5/1
  Delay5/1 -> Product/2
  Product/1 -> Delay/1
  Delay/1 -> Data Type Conversion/1, Relational Operator2/1, Relational Operator1/1
  Delay8/1 -> Product/1
  Delay7/1 -> Data Type Conversion1/1
  Delay9/1 -> Delay1/1
  n_init_assert_out/1 -> Delay12/1
  Delay12/1 -> Delay13/1
  Delay13/1 -> Logical Operator/2
  DataValid/1 -> Delay15/1
  Delay15/1 -> Delay16/1
  Delay16/1 -> Logical Operator/1
  Logical Operator/1 -> Delay14/1
  Delay14/1 -> valid_out/1
  Data Type Conversion1/1 -> Delay6/1
  Delay18/1 -> Delay19/1
  Delay17/1 -> Delay18/1
  data_in/1 -> Delay17/1
  Delay19/1 -> data_out/1, DebugScope/4
  Delay11/1 -> ratio_out/1, DebugScope/2
  Delay6/1 -> energy_out/1, DebugScope/1
  adp_end_threshold_in/1 -> Delay21/1
  Delay21/1 -> Relational Operator2/2
  Relational Operator2/1 -> Delay22/1
  Delay2/1 -> TriggerStateMachine/2(Adp_Trg)  "Adp_Trg"
  Delay22/1 -> TriggerStateMachine/3(Adp_End_Trig)  "Adp_End_Trig"
  TriggerStateMachine/1(StartTrigger) -> DebugScope/3
  TriggerStateMachine/2(TriggerOut) -> trigger_out/1
  [Fix_Trg] -> TriggerStateMachine/1(Fix_Trg)

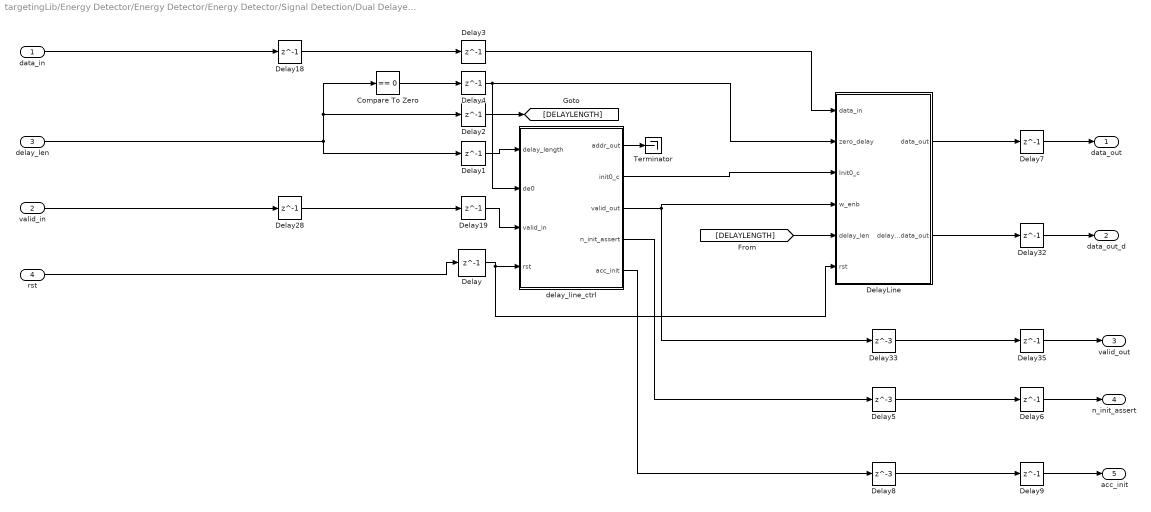
== system targetingLib/Energy Detector/Energy Detector/Energy Detector/Signal Detection/Dual Delayer/Variable Delayer0 ==
  data_in : Inport
  valid_in : Inport  Port=2
  delay_len : Inport  Port=3
  rst : Inport  Port=4
  Compare To Zero : hdlsllib/Logic and Bit Operations/Compare To Zero  relop===  OutDataTypeStr=boolean
  Delay{,1..4,6..7,9,18..19,28,32,35} (13 alike) : Delay  DelayLength=1
  Delay33 : Delay  DelayLength=3
  Delay5 : Delay  DelayLength=3
  Delay8 : Delay  DelayLength=3
  DelayLine : Subsystem
  Terminator : Terminator
  delay_line_ctrl : MATLAB Function  TreatAsAtomicUnit=on
  data_out : Outport
  data_out_d : Outport  Port=2
  valid_out : Outport  Port=3
  n_init_assert : Outport  Port=4
  acc_init : Outport  Port=5
  wires:
  Delay9/1 -> acc_init/1
  Delay8/1 -> Delay9/1
  delay_line_ctrl/5(acc_init) -> Delay8/1
  Delay7/1 -> data_out/1
  DelayLine/1(data_out) -> Delay7/1
  Delay6/1 -> n_init_assert/1
  Delay5/1 -> Delay6/1
  delay_line_ctrl/4(n_init_assert) -> Delay5/1
  DelayLine/2(delayed_data_out) -> Delay32/1
  Delay4/1 -> delay_line_ctrl/2(de0), DelayLine/2(zero_delay)
  Compare To Zero/1 -> Delay4/1
  [DELAYLENGTH] -> DelayLine/5(delay_len)
  Delay18/1 -> Delay3/1
  Delay32/1 -> data_out_d/1
  valid_in/1 -> Delay28/1
  delay_line_ctrl/1(addr_out) -> Terminator/1
  data_in/1 -> Delay18/1
  Delay35/1 -> valid_out/1
  delay_line_ctrl/3(valid_out) -> DelayLine/4(w_enb), Delay33/1
  delay_len/1 -> Compare To Zero/1, Delay2/1, Delay1/1
  Delay3/1 -> DelayLine/1(data_in)
  Delay28/1 -> Delay19/1
  Delay33/1 -> Delay35/1
  delay_line_ctrl/2(init0_c) -> DelayLine/3(Init0_c)
  rst/1 -> Delay/1
  Delay/1 -> delay_line_ctrl/4(rst), DelayLine/6(rst)
  Delay19/1 -> delay_line_ctrl/3(valid_in)
  Delay1/1 -> delay_line_ctrl/1(delay_length)
  Delay2/1 -> [DELAYLENGTH]

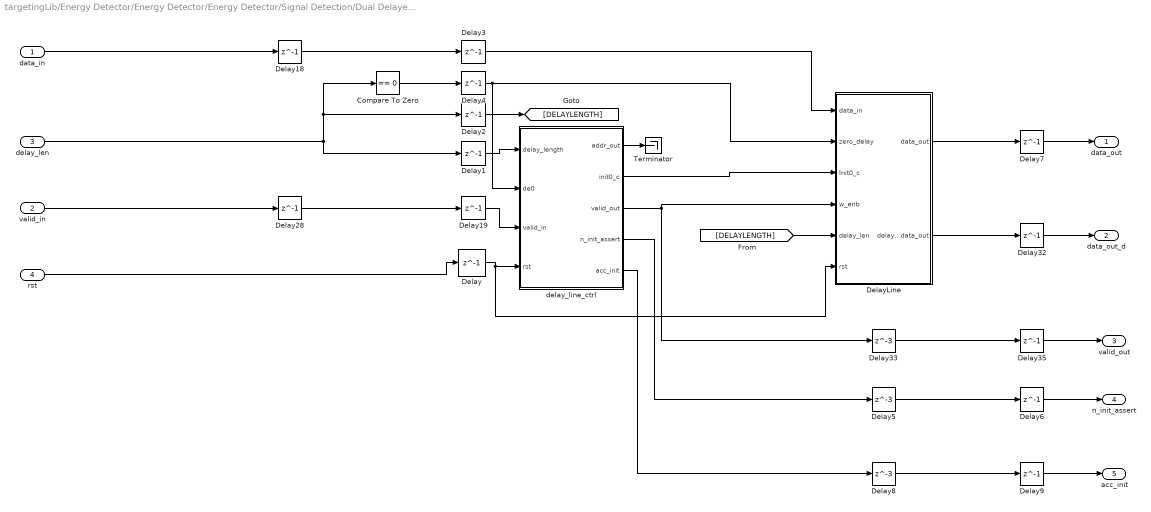
== system targetingLib/Energy Detector/Energy Detector/Energy Detector/Signal Detection/Dual Delayer/Variable Delayer1 ==
  data_in : Inport
  valid_in : Inport  Port=2
  delay_len : Inport  Port=3
  rst : Inport  Port=4
  Compare To Zero : hdlsllib/Logic and Bit Operations/Compare To Zero  relop===  OutDataTypeStr=boolean
  Delay{,1..4,6..7,9,18..19,28,32,35} (13 alike) : Delay  DelayLength=1
  Delay33 : Delay  DelayLength=3
  Delay5 : Delay  DelayLength=3
  Delay8 : Delay  DelayLength=3
  DelayLine : Subsystem
  Terminator : Terminator
  delay_line_ctrl : MATLAB Function  TreatAsAtomicUnit=on
  data_out : Outport
  data_out_d : Outport  Port=2
  valid_out : Outport  Port=3
  n_init_assert : Outport  Port=4
  acc_init : Outport  Port=5
  wires:
  Delay9/1 -> acc_init/1
  Delay8/1 -> Delay9/1
  delay_line_ctrl/5(acc_init) -> Delay8/1
  Delay7/1 -> data_out/1
  DelayLine/1(data_out) -> Delay7/1
  Delay6/1 -> n_init_assert/1
  Delay5/1 -> Delay6/1
  delay_line_ctrl/4(n_init_assert) -> Delay5/1
  DelayLine/2(delayed_data_out) -> Delay32/1
  Delay4/1 -> delay_line_ctrl/2(de0), DelayLine/2(zero_delay)
  Compare To Zero/1 -> Delay4/1
  [DELAYLENGTH] -> DelayLine/5(delay_len)
  Delay18/1 -> Delay3/1
  Delay32/1 -> data_out_d/1
  valid_in/1 -> Delay28/1
  delay_line_ctrl/1(addr_out) -> Terminator/1
  data_in/1 -> Delay18/1
  Delay35/1 -> valid_out/1
  delay_line_ctrl/3(valid_out) -> DelayLine/4(w_enb), Delay33/1
  delay_len/1 -> Compare To Zero/1, Delay2/1, Delay1/1
  Delay3/1 -> DelayLine/1(data_in)
  Delay28/1 -> Delay19/1
  Delay33/1 -> Delay35/1
  delay_line_ctrl/2(init0_c) -> DelayLine/3(Init0_c)
  rst/1 -> Delay/1
  Delay/1 -> delay_line_ctrl/4(rst), DelayLine/6(rst)
  Delay19/1 -> delay_line_ctrl/3(valid_in)
  Delay1/1 -> delay_line_ctrl/1(delay_length)
  Delay2/1 -> [DELAYLENGTH]

== system targetingLib/Energy Detector/Energy Detector/Energy Detector/Signal Detection/Energy Accumulator/DIV0 ==
  N : Inport
  D : Inport  Port=2
  Delay4 : Delay  DelayLength=33
  Delay5 : Delay  DelayLength=1
  Delay6 : Delay  DelayLength=1
  Divide : Product  Inputs=*/
  Q : Outport
  wires:
  D/1 -> Delay6/1
  N/1 -> Delay5/1
  Delay4/1 -> Q/1
  Delay6/1 -> Divide/2
  Delay5/1 -> Divide/1
  Divide/1 -> Delay4/1

== system targetingLib/Energy Detector/Energy Detector/Energy Detector/Signal Detection/Energy Accumulator/ED ACC ==
  data_in : Inport
  delay_data_in : Inport  Port=2
  E : Inport  Port=3
  InitEnb : Inport  Port=4
  R : Inport  Port=5
  Add : Sum  Inputs=+-  OutDataTypeStr=fixdt(1,45,30)
  Data Type Conversion : DataTypeConversion  OutDataTypeStr=fixdt(1,45,30)  SaturateOnIntegerOverflow=off  RndMeth=Floor
  Delay1 : Delay  DelayLength=1
  Delay2 : Delay  DelayLength=1
  Delay3 : Delay  DelayLength=1
  Delay4 : Delay  DelayLength=8
  Delay5 : Delay  DelayLength=8
  Delay6 : Delay  DelayLength=8
  Pow : Subsystem
  Pow1 : Subsystem
  WT Accumulator : Subsystem  TreatAsAtomicUnit=on  mask{totalBitwidth=bitwidth, lowerBitwidth=bitwdith_low}
      mask prompts: totalBitwidth "Accumulator Bitwidth"; lowerBitwidth "Lower Bitwitch"
  acc_out : Outport
  wires:
  Pow/1(DataOut) -> Delay2/1
  E/1 -> Delay6/1
  Add/1 -> Delay3/1
  InitEnb/1 -> Delay4/1
  Delay1/1 -> Add/2
  delay_data_in/1 -> Pow1/1(DataIn)
  data_in/1 -> Pow/1(DataIn)
  Delay3/1 -> WT Accumulator/3(DataIn), WT Accumulator/4(InitDataIn)
  Delay2/1 -> Add/1
  WT Accumulator/1(DataOut) -> Data Type Conversion/1
  R/1 -> Delay5/1
  Pow1/1(DataOut) -> Delay1/1
  Delay4/1 -> WT Accumulator/5(InitEnb)
  Delay5/1 -> WT Accumulator/2(R)
  Delay6/1 -> WT Accumulator/1(E)
  Data Type Conversion/1 -> acc_out/1

== system targetingLib/Energy Detector/Energy Detector/Energy Detector/Signal Detection/Energy Accumulator/ED ACC1 ==
  data_in : Inport
  delay_data_in : Inport  Port=2
  E : Inport  Port=3
  InitEnb : Inport  Port=4
  R : Inport  Port=5
  Add : Sum  Inputs=+-  OutDataTypeStr=fixdt(1,45,30)
  Data Type Conversion : DataTypeConversion  OutDataTypeStr=fixdt(1,45,30)  SaturateOnIntegerOverflow=off  RndMeth=Floor
  Delay1 : Delay  DelayLength=1
  Delay2 : Delay  DelayLength=1
  Delay3 : Delay  DelayLength=1
  Delay4 : Delay  DelayLength=8
  Delay5 : Delay  DelayLength=8
  Delay6 : Delay  DelayLength=8
  Pow : Subsystem
  Pow1 : Subsystem
  WT Accumulator : Subsystem  TreatAsAtomicUnit=on  mask{totalBitwidth=bitwidth, lowerBitwidth=bitwdith_low}
      mask prompts: totalBitwidth "Accumulator Bitwidth"; lowerBitwidth "Lower Bitwitch"
  acc_out : Outport
  wires:
  Pow/1(DataOut) -> Delay2/1
  E/1 -> Delay6/1
  Add/1 -> Delay3/1
  InitEnb/1 -> Delay4/1
  Delay1/1 -> Add/2
  delay_data_in/1 -> Pow1/1(DataIn)
  data_in/1 -> Pow/1(DataIn)
  Delay3/1 -> WT Accumulator/3(DataIn), WT Accumulator/4(InitDataIn)
  Delay2/1 -> Add/1
  WT Accumulator/1(DataOut) -> Data Type Conversion/1
  R/1 -> Delay5/1
  Pow1/1(DataOut) -> Delay1/1
  Delay4/1 -> WT Accumulator/5(InitEnb)
  Delay5/1 -> WT Accumulator/2(R)
  Delay6/1 -> WT Accumulator/1(E)
  Data Type Conversion/1 -> acc_out/1

== system targetingLib/Energy Detector/Energy Detector/Energy Detector/Signal Detection/Thresholding/TriggerStateMachine ==
  Fix_Trg : Inport
  Adp_Trg : Inport  Port=2
  Adp_End_Trig : Inport  Port=3
  End_Trigger : Logic  Operator=OR  IconShape=distinctive  AllPortsSameDT=off  OutDataTypeStr=boolean
  NOT : Logic  Operator=NOT  IconShape=distinctive  AllPortsSameDT=off  OutDataTypeStr=boolean
  S-R Flip-Flop : simulink_extras/Flip Flops/S-R Flip-Flop  initial_condition=0
  Start_Trigger : Logic  AllPortsSameDT=off  OutDataTypeStr=boolean
  Terminator : Terminator
  StartTrigger : Outport
  TriggerOut : Outport  Port=2
  wires:
  S-R Flip-Flop/2 -> Terminator/1
  End_Trigger/1 -> S-R Flip-Flop/2  "End_Trigger"
  Fix_Trg/1 -> Start_Trigger/1, NOT/1
  Start_Trigger/1 -> StartTrigger/1, S-R Flip-Flop/1
  Adp_End_Trig/1 -> End_Trigger/2
  Adp_Trg/1 -> Start_Trigger/2
  NOT/1 -> End_Trigger/1
  S-R Flip-Flop/1 -> TriggerOut/1  "TriggerOut"

== system targetingLib/Energy Detector/Energy Detector/Energy Detector/Signal Detection/Dual Delayer/Variable Delayer0/DelayLine ==
  data_in : Inport
  zero_delay : Inport  Port=2
  Init0_c : Inport  Port=3
  w_enb : Inport  Port=4
  delay_len : Inport  Port=5
  rst : Inport  Port=6
  Constant : Constant  OutDataTypeStr=boolean  SampleTime=-1
  Delay{1,20,23..27,30,36} (9 alike) : Delay  DelayLength=1
  FIFO W Counter1 : hdlsllib/Sources/HDL Counter  CountType=Free running  CountInit=0  CountStep=1  CountMax=25  CountFromType=Initial value  CountFrom=0  CountResetPort=on  CountLoadPort=off  CountEnbPort=on  CountDirPort=off  CountHitOutputPort=off  CountDataType=Unsigned  CountWordLen=depth  CountFracLen=0  CountSampTime=1
  Logical Operator : Logic  Operator=NOT  IconShape=distinctive  AllPortsSameDT=off  OutDataTypeStr=boolean
  Simple Dual Port RAM : hdlsllib/HDL RAMs/Simple Dual Port RAM  ram_size=depth
  Sum1 : Sum  Inputs=+-|  OutDataTypeStr=Inherit: Same as accumulator
  Switch : Switch  Criteria=u2 ~= 0  SaturateOnIntegerOverflow=off  InputSameDT=off
  Switch1 : Switch  Criteria=u2 ~= 0  SaturateOnIntegerOverflow=off  InputSameDT=off
  Unit Delay Resettable Synchronous : hdlsllib/Discrete/Unit Delay Resettable Synchronous  InitialCondition=0.0  SampleTime=-1
  data_out : Outport
  delayed_data_out : Outport  Port=2
  wires:
  Unit Delay Resettable Synchronous/1 -> Switch1/3
  Constant/1 -> Unit Delay Resettable Synchronous/2
  Switch/1 -> delayed_data_out/1
  Logical Operator/1 -> Delay27/1
  Delay1/1 -> Switch/3
  rst/1 -> FIFO W Counter1/1
  zero_delay/1 -> Switch/2
  Delay36/1 -> Delay25/1
  Delay24/1 -> Simple Dual Port RAM/2
  w_enb/1 -> FIFO W Counter1/2, Delay26/1
  Delay26/1 -> Simple Dual Port RAM/3
  delay_len/1 -> Sum1/2
  Delay23/1 -> Simple Dual Port RAM/4
  Sum1/1 -> Delay23/1
  data_in/1 -> Delay20/1
  Init0_c/1 -> Logical Operator/1
  Delay25/1 -> Switch/1, data_out/1
  Switch1/1 -> Delay1/1
  Delay20/1 -> Delay36/1, Simple Dual Port RAM/1
  FIFO W Counter1/1 -> Sum1/1, Delay24/1
  Simple Dual Port RAM/1 -> Switch1/1, Unit Delay Resettable Synchronous/1
  Delay30/1 -> Switch1/2
  Delay27/1 -> Delay30/1

== system targetingLib/Energy Detector/Energy Detector/Energy Detector/Signal Detection/Dual Delayer/Variable Delayer1/DelayLine ==
  data_in : Inport
  zero_delay : Inport  Port=2
  Init0_c : Inport  Port=3
  w_enb : Inport  Port=4
  delay_len : Inport  Port=5
  rst : Inport  Port=6
  Constant : Constant  OutDataTypeStr=boolean  SampleTime=-1
  Delay{1,20,23..27,30,36} (9 alike) : Delay  DelayLength=1
  FIFO W Counter1 : hdlsllib/Sources/HDL Counter  CountType=Free running  CountInit=0  CountStep=1  CountMax=25  CountFromType=Initial value  CountFrom=0  CountResetPort=on  CountLoadPort=off  CountEnbPort=on  CountDirPort=off  CountHitOutputPort=off  CountDataType=Unsigned  CountWordLen=depth  CountFracLen=0  CountSampTime=1
  Logical Operator : Logic  Operator=NOT  IconShape=distinctive  AllPortsSameDT=off  OutDataTypeStr=boolean
  Simple Dual Port RAM : hdlsllib/HDL RAMs/Simple Dual Port RAM  ram_size=depth
  Sum1 : Sum  Inputs=+-|  OutDataTypeStr=Inherit: Same as accumulator
  Switch : Switch  Criteria=u2 ~= 0  SaturateOnIntegerOverflow=off  InputSameDT=off
  Switch1 : Switch  Criteria=u2 ~= 0  SaturateOnIntegerOverflow=off  InputSameDT=off
  Unit Delay Resettable Synchronous : hdlsllib/Discrete/Unit Delay Resettable Synchronous  InitialCondition=0.0  SampleTime=-1
  data_out : Outport
  delayed_data_out : Outport  Port=2
  wires:
  Unit Delay Resettable Synchronous/1 -> Switch1/3
  Constant/1 -> Unit Delay Resettable Synchronous/2
  Switch/1 -> delayed_data_out/1
  Logical Operator/1 -> Delay27/1
  Delay1/1 -> Switch/3
  rst/1 -> FIFO W Counter1/1
  zero_delay/1 -> Switch/2
  Delay36/1 -> Delay25/1
  Delay24/1 -> Simple Dual Port RAM/2
  w_enb/1 -> FIFO W Counter1/2, Delay26/1
  Delay26/1 -> Simple Dual Port RAM/3
  delay_len/1 -> Sum1/2
  Delay23/1 -> Simple Dual Port RAM/4
  Sum1/1 -> Delay23/1
  Init0_c/1 -> Logical Operator/1
  Delay25/1 -> Switch/1, data_out/1
  Switch1/1 -> Delay1/1
  Delay20/1 -> Delay36/1, Simple Dual Port RAM/1
  FIFO W Counter1/1 -> Sum1/1, Delay24/1
  Simple Dual Port RAM/1 -> Switch1/1, Unit Delay Resettable Synchronous/1
  Delay30/1 -> Switch1/2
  Delay27/1 -> Delay30/1
  data_in/1 -> Delay20/1

== system targetingLib/Energy Detector/Energy Detector/Energy Detector/Signal Detection/Energy Accumulator/ED ACC/Pow ==
  DataIn : Inport
  Add : Sum
  Complex to Real-Imag : ComplexToRealImag
  Delay{,1..4,7} (6 alike) : Delay  InitialCondition=0  UseCircularBuffer=on
  Delay5 : Delay  DelayLength=1  InitialCondition=0  UseCircularBuffer=on
  Delay6 : Delay  DelayLength=1  InitialCondition=0  UseCircularBuffer=on
  Delay8 : Delay  DelayLength=1  InitialCondition=0  UseCircularBuffer=on
  Mul : Product  Inputs=**
  Mul1 : Product  Inputs=**
  DataOut : Outport
  wires:
  Delay4/1 -> Delay6/1
  Delay8/1 -> DataOut/1
  Delay5/1 -> Add/2
  Delay2/1 -> Mul1/2
  Mul/1 -> Delay4/1
  Delay7/1 -> Delay2/1, Delay3/1
  DataIn/1 -> Complex to Real-Imag/1
  Delay/1 -> Mul/2
  Add/1 -> Delay8/1
  Delay6/1 -> Add/1
  Complex to Real-Imag/2 -> Delay7/1
  Delay1/1 -> Mul/1
  Complex to Real-Imag/1 -> Delay1/1, Delay/1
  Mul1/1 -> Delay5/1
  Delay3/1 -> Mul1/1

== system targetingLib/Energy Detector/Energy Detector/Energy Detector/Signal Detection/Energy Accumulator/ED ACC/Pow1 ==
  DataIn : Inport
  Add : Sum
  Complex to Real-Imag : ComplexToRealImag
  Delay{,1..4,7} (6 alike) : Delay  InitialCondition=0  UseCircularBuffer=on
  Delay5 : Delay  DelayLength=1  InitialCondition=0  UseCircularBuffer=on
  Delay6 : Delay  DelayLength=1  InitialCondition=0  UseCircularBuffer=on
  Delay8 : Delay  DelayLength=1  InitialCondition=0  UseCircularBuffer=on
  Mul : Product  Inputs=**
  Mul1 : Product  Inputs=**
  DataOut : Outport
  wires:
  Delay4/1 -> Delay6/1
  Delay8/1 -> DataOut/1
  Delay5/1 -> Add/2
  Delay2/1 -> Mul1/2
  Mul/1 -> Delay4/1
  Delay7/1 -> Delay2/1, Delay3/1
  DataIn/1 -> Complex to Real-Imag/1
  Delay/1 -> Mul/2
  Add/1 -> Delay8/1
  Delay6/1 -> Add/1
  Complex to Real-Imag/2 -> Delay7/1
  Delay1/1 -> Mul/1
  Complex to Real-Imag/1 -> Delay1/1, Delay/1
  Mul1/1 -> Delay5/1
  Delay3/1 -> Mul1/1

== system targetingLib/Energy Detector/Energy Detector/Energy Detector/Signal Detection/Energy Accumulator/ED ACC/WT Accumulator ==
  E : Inport
  R : Inport  Port=2
  DataIn : Inport  Port=3
  InitDataIn : Inport  Port=4
  InitEnb : Inport  Port=5
  AccHigh : Subsystem
  AccLow : Subsystem
  Bit Concat : hdlsllib/Logic and Bit Operations/Bit Concat  numInputs=2
  Bit Slice1 : hdlsllib/Logic and Bit Operations/Bit Slice  lidx=totalBitwidth-1  ridx=lowerBitwidth
  Bit Slice2 : hdlsllib/Logic and Bit Operations/Bit Slice  lidx=lowerBitwidth-1  ridx=0
  Bit Slice4 : hdlsllib/Logic and Bit Operations/Bit Slice  lidx=totalBitwidth-1  ridx=lowerBitwidth
  Bit Slice5 : hdlsllib/Logic and Bit Operations/Bit Slice  lidx=lowerBitwidth-1  ridx=0
  Data Type Propagation : sl_signal_attributes/Data Type Propagation  PropDataType=fixdt(1, 16)  IfRefDouble=double  IfRefSingle=single  IsSigned=IsSigned1  NumBitsBase=NumBits2  NumBitsMult=1  NumBitsAdd=0  NumBitsAllowFinal=-1  PropScaling=2^-10  ValuesUsedBestPrec=[5 -7]  SlopeBase=min([Slope1 Slope2])  SlopeMult=1  SlopeAdd=0  BiasBase=Bias1  BiasMult=1  BiasAdd=0
  Data Type Conversion : DataTypeConversion  ConvertRealWorld=Stored Integer (SI)  SaturateOnIntegerOverflow=off  RndMeth=Floor
  Delay{,1..5} (6 alike) : Delay  DelayLength=1
  DataOut : Outport  VectorParamsAs1DForOutWhenUnconnected=off
  wires:
  R/1 -> AccLow/4(rst), Delay2/1
  E/1 -> AccLow/3(AccEnb), Delay3/1
  Bit Slice1/1 -> Delay1/1
  Delay/1 -> Bit Concat/2
  Data Type Conversion/1 -> DataOut/1, Data Type Propagation/3
  Bit Concat/1 -> Data Type Conversion/1, Data Type Propagation/2
  InitEnb/1 -> AccLow/2(InitEnb), Delay4/1
  Bit Slice4/1 -> Delay5/1
  Delay3/1 -> AccHigh/3(AccEnb)
  Delay2/1 -> AccHigh/4(rst)
  Delay1/1 -> AccHigh/5(DataIn)
  AccLow/1(CarryOut) -> AccHigh/6(Carry)
  AccHigh/1(AccOut) -> Bit Concat/1
  Bit Slice5/1 -> AccLow/1(InitDataL)
  Bit Slice2/1 -> AccLow/5(DataIn)
  Delay4/1 -> AccHigh/2(InitEnb)
  Delay5/1 -> AccHigh/1(InitDataH)
  AccLow/2(AccOut) -> Delay/1
  InitDataIn/1 -> Bit Slice5/1, Bit Slice4/1
  DataIn/1 -> Data Type Propagation/1, Bit Slice1/1, Bit Slice2/1
